simulink model "Vant2_lqr"  (R2015a)
settings: Solver=ode45  StartTime=0.0  StopTime=inf  FixedStep=10-4  RelTol=1e-3  SampleTimeConstraint=STIndependent
values from neighbouring files (symbols this model uses):
  G = [10.2751 ; 10.2799 ; 0 ;  0 ]    [MIL_lqr_vant2.m]    (also in Vant2_Hinf_withLoad.m = [12.6005 ; 12.609 ; 0 ;  0 ])
  K = zeros(m,n)    [MIL_lqr_vant2.m]    (also in Vant2_Hinf_withLoad.m)
  T = 0.012    [MIL_lqr_vant2.m]    (also in Vant2_Hinf_withLoad.m)
  Xinit = zeros(n,1)    [MIL_lqr_vant2.m]    (also in Vant2_Hinf_withLoad.m)
  Xref = zeros(n,1)    [MIL_lqr_vant2.m]    (also in Vant2_Hinf_withLoad.m)
libraries: robotlib x8
settings Model: Creator=rblan  LastModifiedBy=rblan

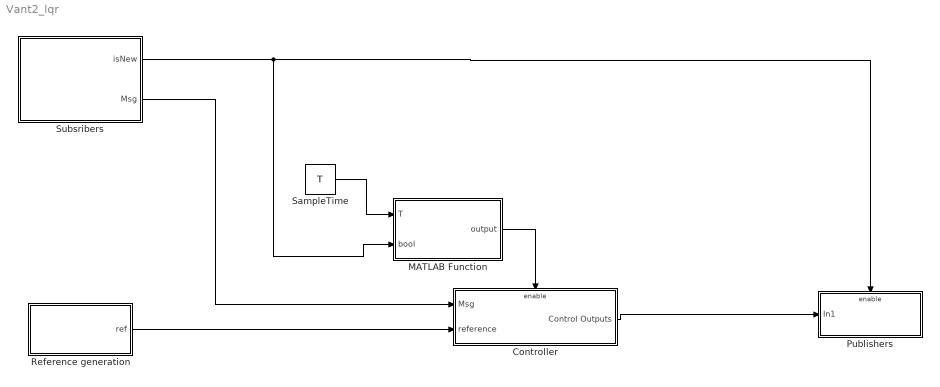
== system Vant2_lqr ==
  Controller : Subsystem
  MATLAB Function : MATLAB Function  TreatAsAtomicUnit=on
  "Publishers " : Subsystem  TreatAsAtomicUnit=on
  "Reference generation " : Subsystem
  SampleTime : Constant  Value=T
  Subsribers : Subsystem
  wires:
  SampleTime/1 -> MATLAB Function/1(T)
  Controller/1(Control Outputs) -> "Publishers "/1(In1)
  Subsribers/2(Msg) -> Controller/1(Msg)
  Subsribers/1(isNew) -> "Publishers "/Enable, MATLAB Function/2(bool)
  "Reference generation "/1("ref ") -> Controller/2(reference)
  MATLAB Function/1(output) -> Controller/Enable

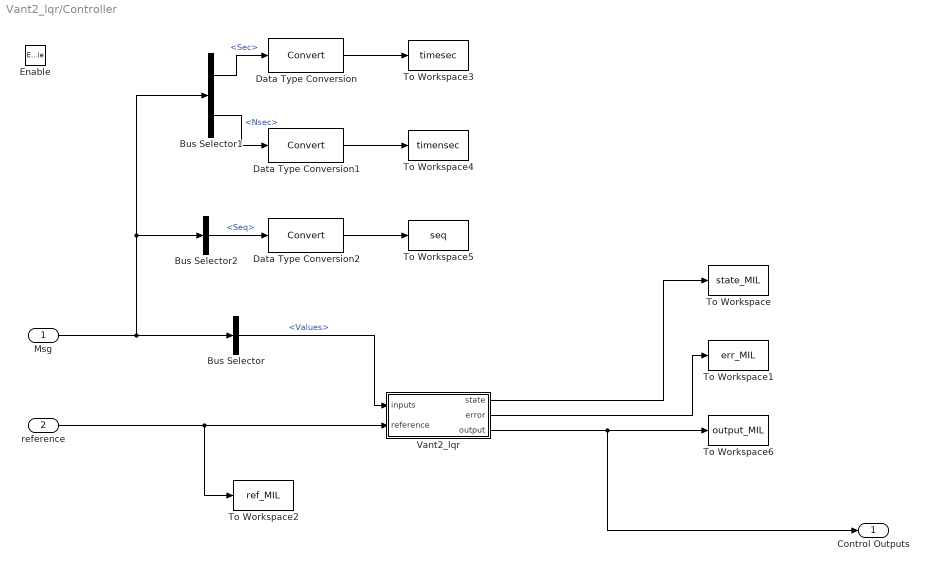
== system Vant2_lqr/Controller ==
  Msg : Inport
  reference : Inport  Port=2
  Enable : EnablePort
  Bus Selector : BusSelector  OutputSignals=Values
  Bus Selector1 : BusSelector  OutputSignals=Header.Stamp.Sec,Header.Stamp.Nsec
  Bus Selector2 : BusSelector  OutputSignals=Header.Seq
  Data Type Conversion : DataTypeConversion
  Data Type Conversion1 : DataTypeConversion
  Data Type Conversion2 : DataTypeConversion
  To Workspace : ToWorkspace  VariableName=state_MIL  SampleTime=-1
  To Workspace1 : ToWorkspace  VariableName=err_MIL  SampleTime=-1
  To Workspace2 : ToWorkspace  VariableName=ref_MIL  SampleTime=-1
  To Workspace3 : ToWorkspace  VariableName=timesec  SampleTime=-1
  To Workspace4 : ToWorkspace  VariableName=timensec  SampleTime=-1
  To Workspace5 : ToWorkspace  VariableName=seq  SampleTime=-1
  To Workspace6 : ToWorkspace  VariableName=output_MIL  SampleTime=-1
  Vant2_lqr : Subsystem
  Control Outputs : Outport
  wires:
  Bus Selector1/2 -> Data Type Conversion1/1  "<Nsec>"
  Bus Selector1/1 -> Data Type Conversion/1  "<Sec>"
  Bus Selector2/1 -> Data Type Conversion2/1  "<Seq>"
  Msg/1 -> Bus Selector2/1, Bus Selector1/1, Bus Selector/1
  Data Type Conversion/1 -> To Workspace3/1
  Data Type Conversion1/1 -> To Workspace4/1
  Data Type Conversion2/1 -> To Workspace5/1
  Bus Selector/1 -> Vant2_lqr/1(inputs)  "<Values>"
  Vant2_lqr/1(state) -> To Workspace/1
  Vant2_lqr/2("error ") -> To Workspace1/1
  Vant2_lqr/3(output) -> To Workspace6/1, Control Outputs/1
  reference/1 -> To Workspace2/1, Vant2_lqr/2(reference)

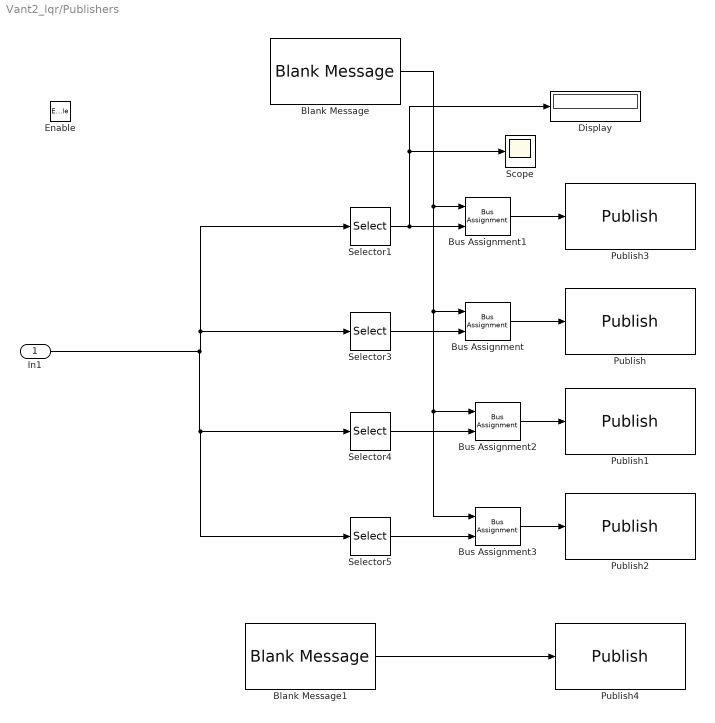
== system Vant2_lqr/Publishers  ==
  In1 : Inport
  Enable : EnablePort
  Blank Message : robotlib/Blank Message  SourceLibraryInfo=This block requires Robotics System Toolbox  messageType=std_msgs/Float64  SampleTime=inf
  Blank Message1 : robotlib/Blank Message  SourceLibraryInfo=This block requires Robotics System Toolbox  messageType=std_msgs/String  SampleTime=inf
  Bus Assignment{,1..3} (4 alike) : BusAssignment  AssignedSignals=Data
  Display : Display
  Publish : robotlib/Publish  SourceLibraryInfo=This block requires Robotics System Toolbox  topicSource=Select from ROS network  topic=/Thrustesq  messageType=std_msgs/Float64  messageQueueLength=1
  Publish1 : robotlib/Publish  SourceLibraryInfo=This block requires Robotics System Toolbox  topicSource=Select from ROS network  topic=/RefaR  messageType=std_msgs/Float64  messageQueueLength=1
  Publish2 : robotlib/Publish  SourceLibraryInfo=This block requires Robotics System Toolbox  topicSource=Select from ROS network  topic=/RefaL  messageType=std_msgs/Float64  messageQueueLength=1
  Publish3 : robotlib/Publish  SourceLibraryInfo=This block requires Robotics System Toolbox  topicSource=Select from ROS network  topic=/Thrustdir  messageType=std_msgs/Float64  messageQueueLength=1
  Publish4 : robotlib/Publish  SourceLibraryInfo=This block requires Robotics System Toolbox  topicSource=Select from ROS network  topic=/Step  messageType=std_msgs/String  messageQueueLength=1
  Scope : Scope
      settings: YMin=13.87  YMax=13.99
  Selector1 : Selector  InputPortWidth=4  Indices=[1]
  Selector3 : Selector  InputPortWidth=4  Indices=[2]
  Selector4 : Selector  InputPortWidth=4  Indices=[3]
  Selector5 : Selector  InputPortWidth=4  Indices=[4]
  wires:
  Bus Assignment/1 -> Publish/1
  Bus Assignment1/1 -> Publish3/1
  Bus Assignment2/1 -> Publish1/1
  Bus Assignment3/1 -> Publish2/1
  Blank Message/1 -> Bus Assignment3/1, Bus Assignment2/1, Bus Assignment/1, Bus Assignment1/1
  Selector1/1 -> Display/1, Scope/1, Bus Assignment1/2
  Selector3/1 -> Bus Assignment/2
  Selector4/1 -> Bus Assignment2/2
  Selector5/1 -> Bus Assignment3/2
  In1/1 -> Selector5/1, Selector4/1, Selector3/1, Selector1/1
  Blank Message1/1 -> Publish4/1

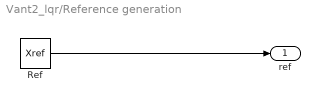
== system Vant2_lqr/Reference generation  ==
  "Ref " : Constant  Value=Xref
  "ref " : Outport
  wires:
  "Ref "/1 -> "ref "/1

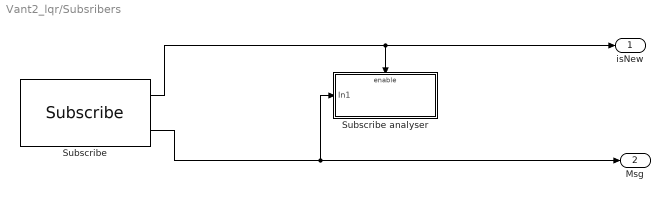
== system Vant2_lqr/Subsribers ==
  Subscribe : robotlib/Subscribe  SourceLibraryInfo=This block requires Robotics System Toolbox  topicSource=Select from ROS network  topic=/Estados  messageType=simulator_msgs/Sensor  sampleTime=-1  messageQueueLength=1
  Subscribe analyser : Subsystem
  isNew : Outport
  Msg : Outport  Port=2
  wires:
  Subscribe/2 -> Msg/1, Subscribe analyser/1(In1)
  Subscribe/1 -> Subscribe analyser/Enable, isNew/1

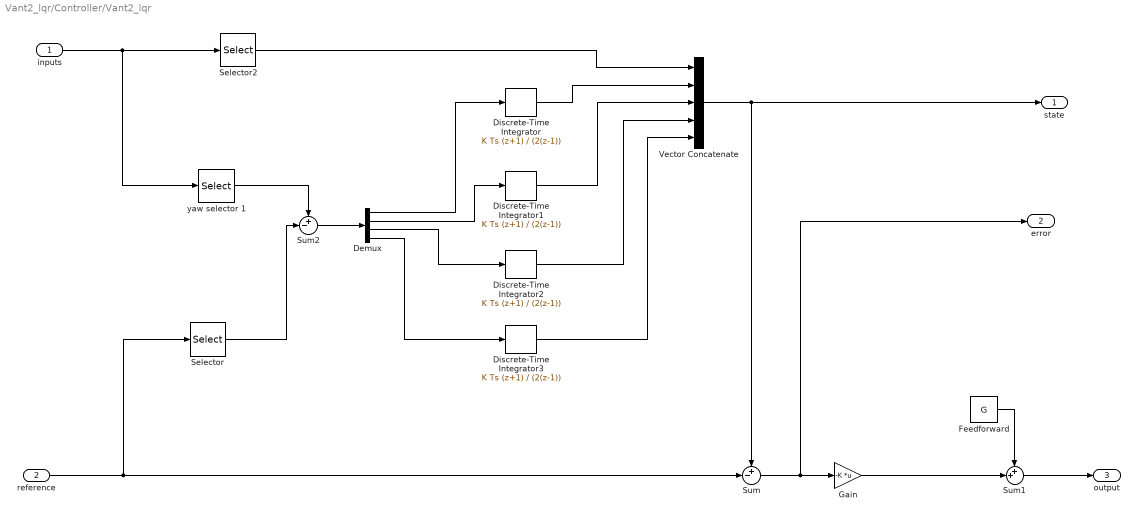
== system Vant2_lqr/Controller/Vant2_lqr ==
  inputs : Inport
  reference : Inport  Port=2
  Demux : Demux
  Discrete-Time Integrator : DiscreteIntegrator  IntegratorMethod=Integration: Trapezoidal  InitialCondition=Xinit(1)  InitialConditionSetting=State (most efficient)  SampleTime=T
  Discrete-Time Integrator1 : DiscreteIntegrator  IntegratorMethod=Integration: Trapezoidal  InitialCondition=Xinit(2)  InitialConditionSetting=State (most efficient)  SampleTime=T
  Discrete-Time Integrator2 : DiscreteIntegrator  IntegratorMethod=Integration: Trapezoidal  InitialCondition=Xinit(3)  InitialConditionSetting=State (most efficient)  SampleTime=T
  Discrete-Time Integrator3 : DiscreteIntegrator  IntegratorMethod=Integration: Trapezoidal  InitialCondition=Xinit(3)  InitialConditionSetting=State (most efficient)  SampleTime=T
  Feedforward : Constant  Value=G
  Gain : Gain  Gain=-K  Multiplication=Matrix(K*u)
  Selector : Selector  InputPortWidth=20  Indices=[1;2;3;6]
  Selector2 : Selector  InputPortWidth=128  Indices=[1; 2; 3; 4; 5; 6; 7; 8; 9;10;11;12;13;14;15;16 ]
  Sum : Sum  Inputs=+-|
  Sum1 : Sum  Inputs=++|
  Sum2 : Sum  Inputs=+-|
  Vector Concatenate : Concatenate  NumInputs=5
  yaw selector 1 : Selector  InputPortWidth=128  Indices=[1;2;3;6]
  state : Outport
  "error " : Outport  Port=2
  output : Outport  Port=3
  wires:
  Discrete-Time Integrator/1 -> Vector Concatenate/2
  Discrete-Time Integrator1/1 -> Vector Concatenate/3
  Discrete-Time Integrator2/1 -> Vector Concatenate/4
  Discrete-Time Integrator3/1 -> Vector Concatenate/5
  Selector2/1 -> Vector Concatenate/1
  Sum/1 -> "error "/1, Gain/1
  Gain/1 -> Sum1/2
  Feedforward/1 -> Sum1/1
  yaw selector 1/1 -> Sum2/1
  Demux/3 -> Discrete-Time Integrator2/1
  Demux/1 -> Discrete-Time Integrator/1
  Demux/2 -> Discrete-Time Integrator1/1
  Demux/4 -> Discrete-Time Integrator3/1
  Selector/1 -> Sum2/2
  Vector Concatenate/1 -> state/1, Sum/1
  Sum2/1 -> Demux/1
  inputs/1 -> yaw selector 1/1, Selector2/1
  reference/1 -> Sum/2, Selector/1
  Sum1/1 -> output/1

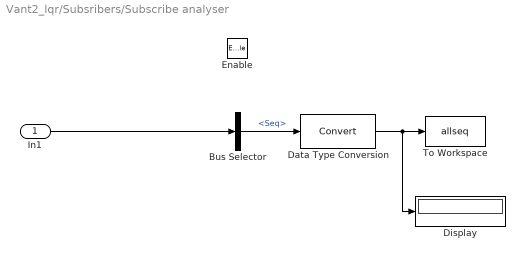
== system Vant2_lqr/Subsribers/Subscribe analyser ==
  In1 : Inport
  Enable : EnablePort
  Bus Selector : BusSelector  OutputSignals=Header.Seq
  Data Type Conversion : DataTypeConversion
  Display : Display
  To Workspace : ToWorkspace  VariableName=allseq  SaveFormat=Timeseries  SampleTime=-1
  wires:
  Bus Selector/1 -> Data Type Conversion/1  "<Seq>"
  Data Type Conversion/1 -> Display/1, To Workspace/1
  In1/1 -> Bus Selector/1

== matlab function Vant2_lqr/MATLAB Function ==
  data: T input; output output; bool input
function output = sampler( T , bool )
%UNTITLED Summary of this function goes here
%   Detailed explanation goes here
persistent decimator ;
if isempty(decimator)
    decimator = 0 ;
end


if (bool == true)

    if mod(decimator,T*1000) == 0
        output = true ;
        decimator=0 ;
    else output = false ;
    end
    decimator=decimator +1 ;
else output = false ;

end


end
